simulink model "Motorized_Pendulum_VSC"  (R2021a)
settings: Solver=ode45  StartTime=0.0  StopTime=tsim  RelTol=1e-9
undefined symbols (not defined in the file): b_n, C_BL, fric_mod, g_n, Jm, Jp, K_n, Ka_fit, KcRa, Km, Kp, Kt, L_n, lambda_n, M_n, N_n, Switch_Law, T_ba_n, Three_Ctrl_Struc, x0
libraries: simulink_extras x2, simulink x1
settings Model: Creator=domin  LastModifiedBy=domin
settings SolverCC: ZeroCrossAlgorithm=Adaptive  AlgebraicLoopSolver=TrustRegion
settings DebuggingCC: IgnoredZcDiagnostic=none  SFMachineParentedDataDiag=warning

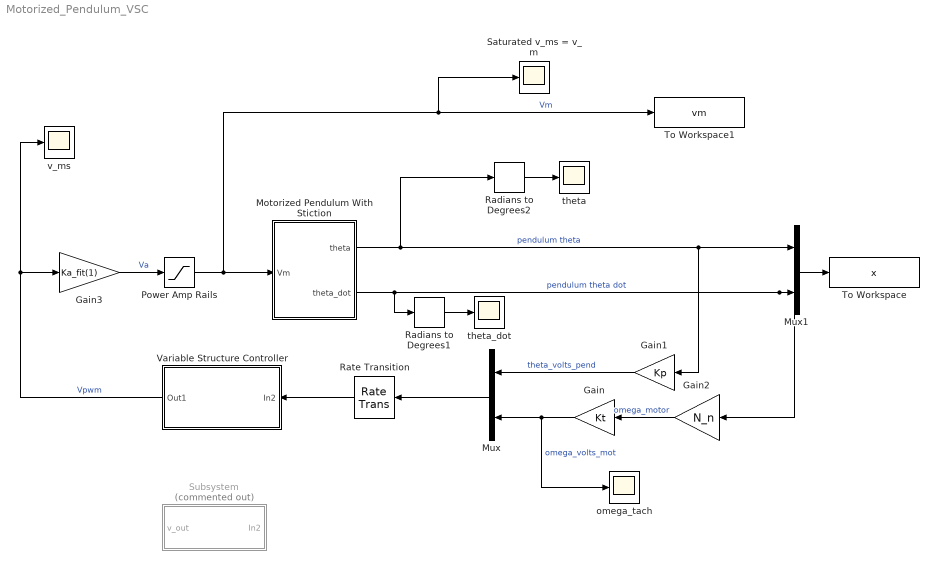
== system Motorized_Pendulum_VSC ==
  Gain : Gain  Gain=Kt
  Gain1 : Gain  Gain=Kp
  Gain2 : Gain  Gain=N_n
  Gain3 : Gain  Gain=Ka_fit(1)
  Motorized Pendulum With Stiction : Subsystem
  Mux : Mux  Inputs=2
  Mux1 : Mux  Inputs=2
  Power Amp Rails : Saturate  UpperLimit=15  LowerLimit=-15
  Radians to Degrees1 : simulink_extras/Transformations/Radians to Degrees
  Radians to Degrees2 : simulink_extras/Transformations/Radians to Degrees
  Rate Transition : RateTransition  OutPortSampleTime=t_samp
  Saturated v_ms = v_m : Scope
  Subsystem : Subsystem  Commented=on
  To Workspace : ToWorkspace  VariableName=x  SampleTime=-1
  To Workspace1 : ToWorkspace  VariableName=vm
  Variable Structure Controller : Subsystem
  omega_tach : Scope
  theta : Scope
  theta_dot : Scope
  v_ms : Scope
  wires:
  Power Amp Rails/1 -> Saturated v_ms = v_m/1, To Workspace1/1, Motorized Pendulum With Stiction/1(Vm)  "Vm"
  Radians to Degrees2/1 -> theta/1
  Variable Structure Controller/1(Out1) -> v_ms/1, Gain3/1  "Vpwm"
  Mux/1 -> Rate Transition/1
  Motorized Pendulum With Stiction/1(theta) -> Radians to Degrees2/1, Gain1/1, Mux1/1  "pendulum theta"
  Motorized Pendulum With Stiction/2(theta_dot) -> Gain2/1, Mux1/2, Radians to Degrees1/1  "pendulum theta dot"
  Rate Transition/1 -> Variable Structure Controller/1(In2)
  Gain2/1 -> Gain/1  "omega_motor"
  Gain/1 -> omega_tach/1, Mux/2  "omega_volts_mot"
  Gain1/1 -> Mux/1  "theta_volts_pend"
  Gain3/1 -> Power Amp Rails/1  "Va"
  Mux1/1 -> To Workspace/1
  Radians to Degrees1/1 -> theta_dot/1

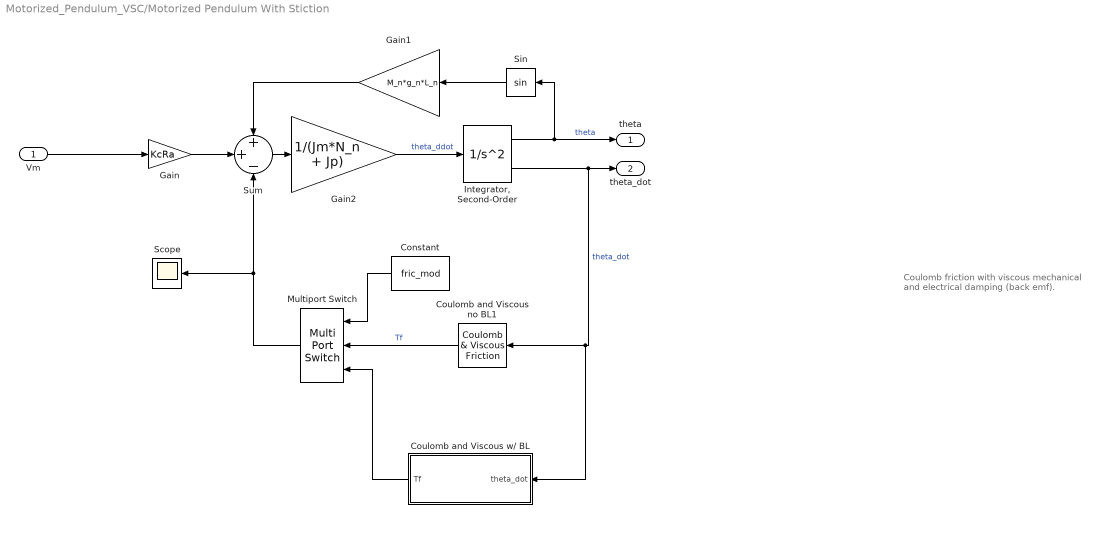
== system Motorized_Pendulum_VSC/Motorized Pendulum With Stiction ==
  note: Coulomb friction with viscous mechanical
      | and electrical damping (back emf).
  Vm : Inport
  Constant : Constant  Value=fric_mod
  Coulomb and Viscous no BL1 : simulink/Discontinuities/Coulomb & Viscous Friction  offset=T_ba_n  gain=N_n*KcRa/Km
  Coulomb and Viscous w/ BL : MATLAB Function  TreatAsAtomicUnit=on
  Gain : Gain  Gain=KcRa
  Gain1 : Gain  Gain=M_n*g_n*L_n
  Gain2 : Gain  Gain=1/(Jm*N_n + Jp)
  "Integrator, Second-Order" : SecondOrderIntegrator  ICX=x0(1)  ICDXDT=x0(2)  ZeroCross=off
  Multiport Switch : MultiPortSwitch  Inputs=2
  Scope : Scope
  Sin : Trigonometry
  Sum : Sum  Inputs=++-
  theta : Outport
  theta_dot : Outport  Port=2
  wires:
  Gain2/1 -> "Integrator, Second-Order"/1  "theta_ddot"
  Sin/1 -> Gain1/1
  "Integrator, Second-Order"/1 -> Sin/1, theta/1  "theta"
  Gain1/1 -> Sum/1
  Sum/1 -> Gain2/1
  Vm/1 -> Gain/1
  Gain/1 -> Sum/2
  "Integrator, Second-Order"/2 -> Coulomb and Viscous w/ BL/1(theta_dot), Coulomb and Viscous no BL1/1, theta_dot/1  "theta_dot"
  Coulomb and Viscous w/ BL/1(Tf) -> Multiport Switch/3
  Coulomb and Viscous no BL1/1 -> Multiport Switch/2  "Tf"
  Constant/1 -> Multiport Switch/1
  Multiport Switch/1 -> Sum/3, Scope/1

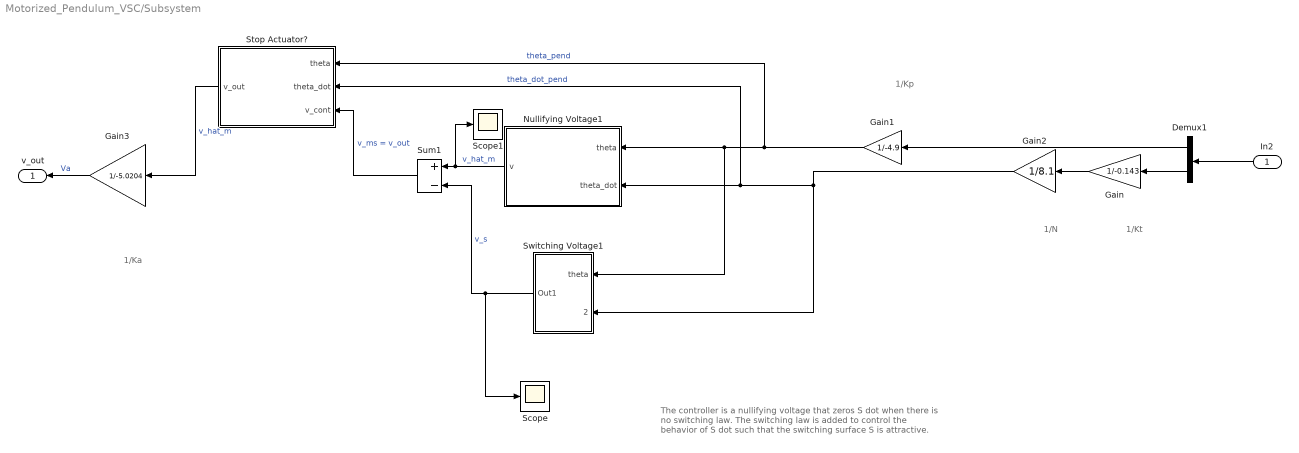
== system Motorized_Pendulum_VSC/Subsystem ==
  note: 1/Kt
  note: 1/N
  note: 1/Ka
  note: 1/Kp
  note: The controller is a nullifying voltage that zeros S dot
      | when there is no switching law. The switching law is added
      | to control the behavior of S dot such that the switching surface
      | S is attractive.
  In2 : Inport  SampleTime=.01
  Demux1 : Demux  Outputs=2
  Gain : Gain  Gain=1/-0.143
  Gain1 : Gain  Gain=1/-4.9
  Gain2 : Gain  Gain=1/8.1
  Gain3 : Gain  Gain=1/-5.0204
  Nullifying Voltage1 : MATLAB Function  TreatAsAtomicUnit=on
  Scope : Scope
  Scope1 : Scope
  Stop Actuator? : MATLAB Function  TreatAsAtomicUnit=on
  Sum1 : Sum  Inputs=+-
  Switching Voltage1 : Subsystem
  v_out : Outport  SampleTime=0
  wires:
  Gain3/1 -> v_out/1  "Va"
  Gain1/1 -> Stop Actuator?/1(theta), Nullifying Voltage1/1(theta), Switching Voltage1/1(theta)  "theta_pend"
  Gain2/1 -> Switching Voltage1/2(theta_dot), Stop Actuator?/2(theta_dot), Nullifying Voltage1/2(theta_dot)  "theta_dot_pend"
  Gain/1 -> Gain2/1
  Switching Voltage1/1(Out1) -> Scope/1, Sum1/2  "v_s"
  Demux1/2 -> Gain/1
  In2/1 -> Demux1/1
  Sum1/1 -> Stop Actuator?/3(v_cont)  "v_ms = v_out"
  Nullifying Voltage1/1(v) -> Scope1/1, Sum1/1  "v_hat_m"
  Stop Actuator?/1(v_out) -> Gain3/1  "v_hat_m"
  Demux1/1 -> Gain1/1

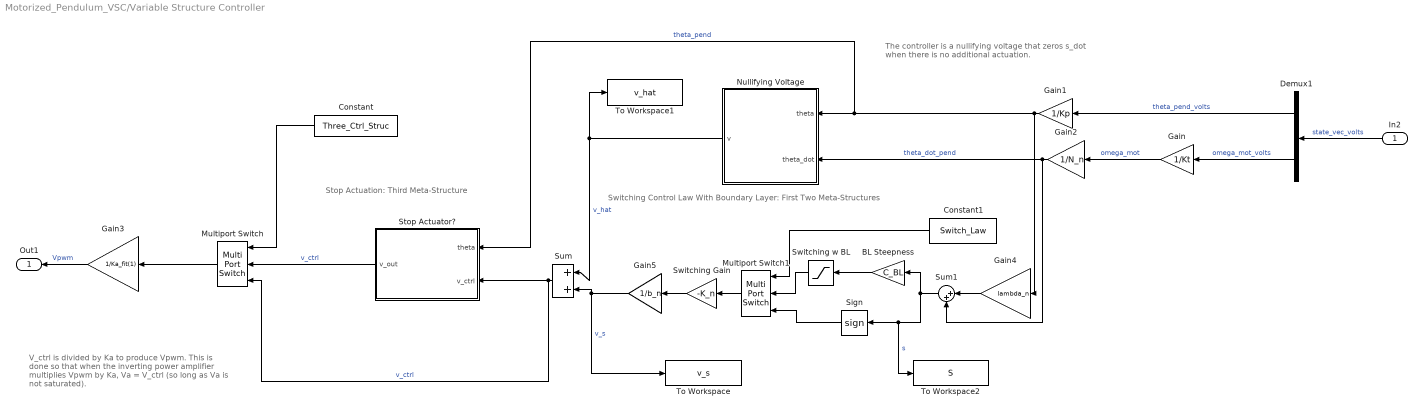
== system Motorized_Pendulum_VSC/Variable Structure Controller ==
  note: Stop Actuation:
      | Third Meta-Structure
  note: Switching Control Law With Boundary Layer: First Two Meta-Structures
  note: V_ctrl is divided by Ka to produce Vpwm. This is
      | done so that when the inverting
      | power amplifier multiplies Vpwm by Ka,
      |  Va = V_ctrl (so long as Va is not saturated).
  note: The controller is a nullifying voltage that zeros s_dot
      | when there is no additional actuation.
  In2 : Inport
  BL Steepness : Gain  Gain=C_BL
  Constant : Constant  Value=Three_Ctrl_Struc
  Constant1 : Constant  Value=Switch_Law
  Demux1 : Demux  Outputs=2
  Gain : Gain  Gain=1/Kt
  Gain1 : Gain  Gain=1/Kp
  Gain2 : Gain  Gain=1/N_n
  Gain3 : Gain  Gain=1/Ka_fit(1)
  Gain4 : Gain  Gain=lambda_n
  Gain5 : Gain  Gain=1/b_n
  Multiport Switch : MultiPortSwitch  Inputs=2
  Multiport Switch1 : MultiPortSwitch  Inputs=2
  Nullifying Voltage : MATLAB Function  TreatAsAtomicUnit=on
  Sign : Signum
  Stop Actuator? : MATLAB Function  TreatAsAtomicUnit=on
  Sum : Sum  Inputs=|++
  Sum1 : Sum  Inputs=|++
  Switching Gain : Gain  Gain=-K_n
  Switching w BL : Saturate  UpperLimit=1  LowerLimit=-1
  To Workspace : ToWorkspace  VariableName=v_s
  To Workspace1 : ToWorkspace  VariableName=v_hat
  To Workspace2 : ToWorkspace  VariableName=S
  Out1 : Outport
  wires:
  Nullifying Voltage/1(v) -> Sum/1, To Workspace1/1  "v_hat"
  Gain1/1 -> Nullifying Voltage/1(theta), Stop Actuator?/1(theta), Gain4/1  "theta_pend"
  Gain2/1 -> Nullifying Voltage/2(theta_dot), Sum1/2  "theta_dot_pend"
  Switching Gain/1 -> Gain5/1
  Sum/1 -> Stop Actuator?/2(v_ctrl), Multiport Switch/3  "v_ctrl"
  In2/1 -> Demux1/1  "state_vec_volts"
  Gain/1 -> Gain2/1  "omega_mot"
  Demux1/2 -> Gain/1  "omega_mot_volts"
  Demux1/1 -> Gain1/1  "theta_pend_volts"
  Gain3/1 -> Out1/1  "Vpwm"
  Gain5/1 -> Sum/2, To Workspace/1  "v_s"
  Gain4/1 -> Sum1/1
  Sum1/1 -> BL Steepness/1, To Workspace2/1, Sign/1  "s"
  BL Steepness/1 -> Switching w BL/1
  Switching w BL/1 -> Multiport Switch1/2
  Stop Actuator?/1(v_out) -> Multiport Switch/2  "v_ctrl"
  Multiport Switch/1 -> Gain3/1
  Constant/1 -> Multiport Switch/1
  Sign/1 -> Multiport Switch1/3
  Multiport Switch1/1 -> Switching Gain/1
  Constant1/1 -> Multiport Switch1/1

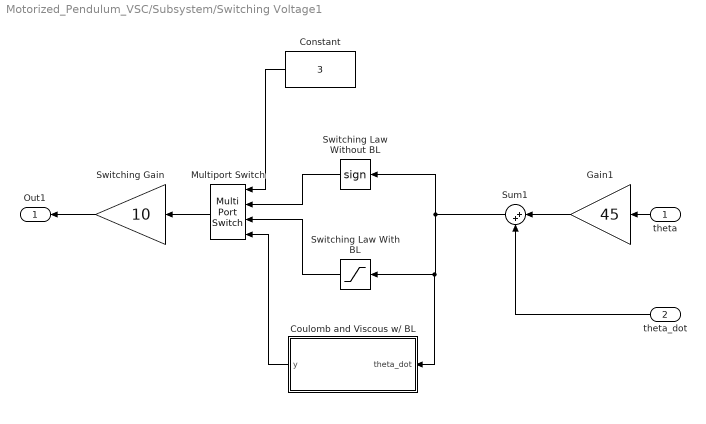
== system Motorized_Pendulum_VSC/Subsystem/Switching Voltage1 ==
  theta : Inport
  theta_dot : Inport  Port=2
  Constant : Constant  Value=3
  Coulomb and Viscous w/ BL : MATLAB Function  TreatAsAtomicUnit=on
  Gain1 : Gain  Gain=45
  Multiport Switch : MultiPortSwitch
  Sum1 : Sum  Inputs=|++
  Switching Gain : Gain  Gain=10
  Switching Law With BL : Saturate  UpperLimit=1  LowerLimit=-1
  Switching Law Without BL : Signum
  Out1 : Outport
  wires:
  Gain1/1 -> Sum1/1
  theta/1 -> Gain1/1
  Switching Gain/1 -> Out1/1
  Sum1/1 -> Coulomb and Viscous w/ BL/1(theta_dot), Switching Law With BL/1, Switching Law Without BL/1
  theta_dot/1 -> Sum1/2
  Constant/1 -> Multiport Switch/1
  Multiport Switch/1 -> Switching Gain/1
  Switching Law Without BL/1 -> Multiport Switch/2
  Switching Law With BL/1 -> Multiport Switch/3
  Coulomb and Viscous w/ BL/1(y) -> Multiport Switch/4

== matlab function Motorized_Pendulum_VSC/Motorized Pendulum With Stiction/Coulomb and Viscous w// BL ==
  data: theta_dot input; Tf output; Km parameter; KcRa parameter; N_n parameter; T_ba_n parameter
function Tf = fcn(theta_dot, Km,  KcRa, N_n, T_ba_n)

Tf = N_n*KcRa/Km*theta_dot + T_ba_n*erf(1e6*theta_dot);

== matlab function Motorized_Pendulum_VSC/Variable Structure Controller/Nullifying Voltage ==
  data: theta input; theta_dot input; v output; lambda_n parameter; K_n parameter
function v = fcn(theta, theta_dot, lambda_n, K_n)


v = 0.3501*theta_dot + 1.0684*sign(theta_dot) - 0.6600*sin(theta_dot)...
    - 0.1144*lambda_n*theta_dot;

% v = 0.3501*theta_dot - 1.0684*sign(theta_dot) - 0.6600*sin(theta_dot)...
%     - 0.1144*lambda_n*theta_dot;

== matlab function Motorized_Pendulum_VSC/Variable Structure Controller/Stop Actuator? ==
  data: theta input; v_out output; v_ctrl input
function v_out = fcn(theta, v_ctrl)

if abs(theta) <=.001
    
    v_out = 0;
    
else
    
    v_out = v_ctrl;
end

== matlab function Motorized_Pendulum_VSC/Subsystem/Nullifying Voltage1 ==
  data: theta input; theta_dot input; v output
function v = fcn(theta, theta_dot)

lambda_n = 45;
v = 0.3501*theta_dot - 1.0684*sign(theta_dot) - 0.6600*sin(theta_dot)...
    - 0.1144*lambda_n*theta_dot;

== matlab function Motorized_Pendulum_VSC/Subsystem/Stop Actuator? ==
  data: theta input; theta_dot input; v_out output; v_cont input
function v_out = fcn(theta, theta_dot, v_cont)

if norm([theta theta_dot])<=.3
    
    v_out = 0;
    
else
    
    v_out = v_cont;
end

== matlab function Motorized_Pendulum_VSC/Subsystem/Switching Voltage1/Coulomb and Viscous w// BL ==
  data: theta_dot input; y output
function y = fcn(theta_dot)

y = erf(1.25*theta_dot);
